simulink model "ASKV3"  (R2024b)
settings: Solver=VariableStepAuto  StartTime=0.0  StopTime=1  RelTol=1e-3
libraries: simulink_extras x3, simulink x3, dspfdesign x1, dspvision x1
settings Model: LastModifiedBy=fredy

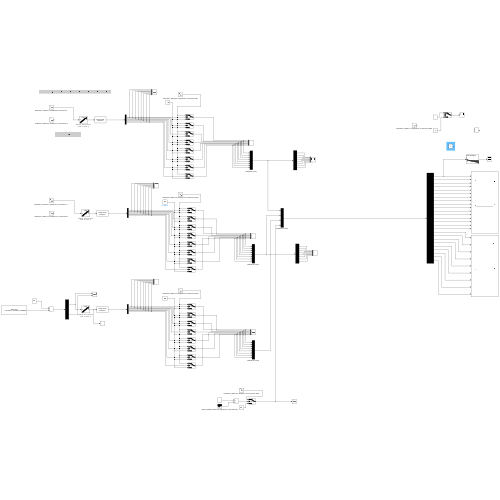
[thumbnail: Simulink's stored preview of the top-level diagram]
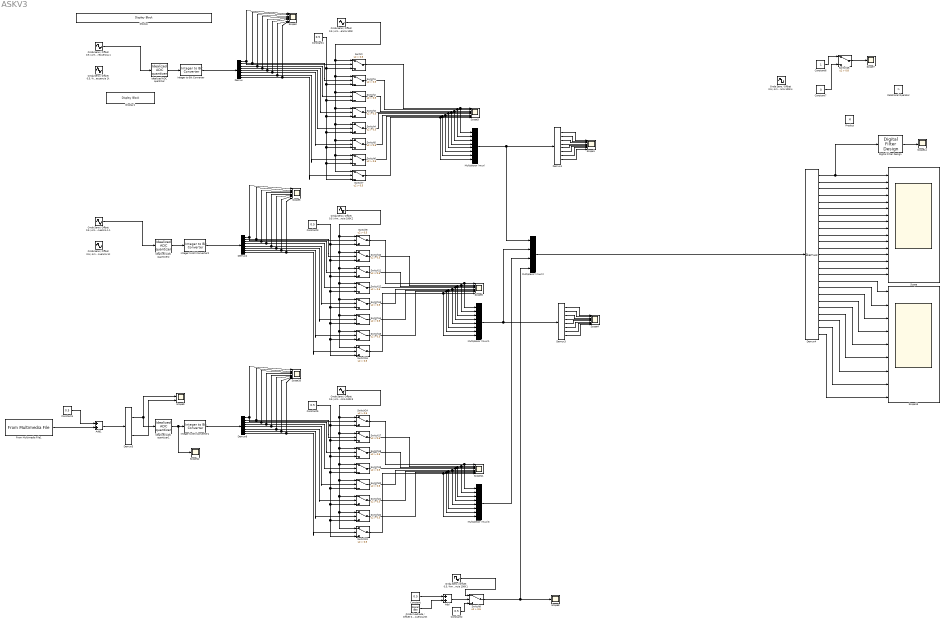
== system ASKV3 ==
  Add : Sum
  Add1 : Sum
  Constant{,1..5} (6 alike) : Constant  Value=0.5
  Constant6 : Constant
  Constant7 : Constant  Value=0
  Demux{,1..3,6} (5 alike) : Demux  Outputs=8
  Demux4 : Demux  Outputs=25
  Demux5 : Demux  Outputs=2
  Digital Filter Design : dspfdesign/Digital Filter Design  mwdsp_browser_bugfix_var=off
  Display : DisplayBlock  LabelPosition=Hide  Transparency=1  Layout=Fill available space
  Display1 : DisplayBlock  LabelPosition=Hide  Transparency=1
  From Multimedia File1 : dspvision/From Multimedia File  inputFilename=D:\Datos Fredy\Programacion\Matlab\Modulacion ASK\audio.mp3  readRange=[1 Inf]  loop=on  numPlays=inf  outputStreams=Audio only  videoDataType=single  audioDataType=single  inheritSampleTime=on  userDefinedSampleTime=1/30  noAudioOutput=off  isIntensityVideo=off  fourcc=RGB  colorVideoFormat=Separate color signals  outputEOF=off  dataOrg=Column-major  audioFrameSize=1  computeAudioFrameSize=off  outSamplingMode=Sample based
      settings: LibrarySourceBlock=audiosources/From Multimedia File
  Idealized ADC quantizer : simulink_extras/Additional Discrete/Idealized ADC quantizer  NumberOfConverterBits=8  Vmin=0  Vmax=1  OutputDataType=double  OutputNegativeValues=off
  Idealized ADC quantizer1 : simulink_extras/Additional Discrete/Idealized ADC quantizer  NumberOfConverterBits=8  Vmin=0  Vmax=1  OutputDataType=double  OutputNegativeValues=off
  Idealized ADC quantizer2 : simulink_extras/Additional Discrete/Idealized ADC quantizer  NumberOfConverterBits=8  Vmin=0  Vmax=1  OutputDataType=double  OutputNegativeValues=off
  Integer to Bit Converter : simulink/Logic and Bit Operations/Integer to Bit Converter  nbits=8  signedInputValues=Unsigned  bitOrder=MSB first  outDtype=Inherit via internal rule
  Integer to Bit Converter1 : simulink/Logic and Bit Operations/Integer to Bit Converter  nbits=8  signedInputValues=Unsigned  bitOrder=MSB first  outDtype=Inherit via internal rule
  Integer to Bit Converter2 : simulink/Logic and Bit Operations/Integer to Bit Converter  nbits=8  signedInputValues=Unsigned  bitOrder=MSB first  outDtype=Inherit via internal rule
  Multiplexor (mux) : Mux  Inputs=8
  Multiplexor (mux)1 : Mux  Inputs=8
  Multiplexor (mux)2 : Mux
  Multiplexor (mux)3 : Mux  Inputs=8
  Onda Cuadrada / Offset 0.5 / Amplitud 0.5 / Frecuencia 5K : SignalGenerator  WaveForm=square  Amplitude=0.5  Frequency=5000
  Onda Seno / Offset 0.5 / Amplitud 0.5 / Frecuencia 1 : Sin  Amplitude=0.5  Bias=0.5  Frequency=6.28321853071  SampleTime=0
  Onda Seno / Offset 0.5 / Amplitud 0.5 / Frecuencia 1.1 : Sin  Amplitude=0.5  Bias=0.5  Frequency=6.28321853071  SampleTime=0
  Onda Seno / Offset 0.5 / Amplitud 0.5 / Frecuencia 100K{,1..4} (5 alike) : Sin  Amplitude=0.5  Bias=0.5  Frequency=628318.5307  SampleTime=0
  Onda Seno / Offset 0.5 / Amplitud 0.5 / Frecuencia 1K : Sin  Amplitude=0.5  Bias=0.5  Frequency=6283.185307  SampleTime=0
  Onda Seno / Offset 0.5 / Amplitud 0.5 / Frecuencia 1k : Sin  Amplitude=0.5  Bias=0.5  Frequency=628321.853071  SampleTime=0
  Product : Product
  Relational Operator : RelationalOperator  Operator=>  OutDataTypeStr=boolean  RndMeth=Simplest  InputSameDT=off
  Scope : Scope  NumInputPorts=16
  Scope{1..6,10..11} (8 alike) : Scope  NumInputPorts=8
  Scope{7..8,12,14} (4 alike) : Scope
  Scope13 : Scope  NumInputPorts=9
  Scope9 : Scope  NumInputPorts=2
  Switch{,1..24} (25 alike) : Switch  Criteria=u2 > Threshold  Threshold=0.5  SaturateOnIntegerOverflow=off  InputSameDT=off
  Switch25 : Switch  Criteria=u2 > Threshold  Threshold=0.8  SaturateOnIntegerOverflow=off  InputSameDT=off
  wires:
  Constant/1 -> Add/1
  Onda Cuadrada / Offset 0.5 / Amplitud 0.5 / Frecuencia 5K/1 -> Add/2
  Add/1 -> Switch8/2
  Idealized ADC quantizer/1 -> Integer to Bit Converter/1
  Onda Seno / Offset 0.5 / Amplitud 0.5 / Frecuencia 100K/1 -> Switch1/1, Switch2/1, Switch7/1, Switch6/1, Switch5/1, Switch4/1, Switch3/1, Switch/1
  Constant1/1 -> Switch/3, Switch1/3, Switch2/3, Switch6/3, Switch7/3, Switch5/3, Switch4/3, Switch3/3
  Idealized ADC quantizer2/1 -> Integer to Bit Converter2/1
  Integer to Bit Converter2/1 -> Demux2/1
  Demux/1 -> Switch/2, Scope2/1
  Integer to Bit Converter/1 -> Demux/1
  Onda Seno / Offset 0.5 / Amplitud 0.5 / Frecuencia 1/1 -> Idealized ADC quantizer/1
  Demux/2 -> Switch1/2, Scope2/2
  Demux/3 -> Switch2/2, Scope2/3
  Demux/5 -> Switch4/2, Scope2/5
  Demux/4 -> Switch3/2, Scope2/4
  Demux/6 -> Switch5/2, Scope2/6
  Demux/7 -> Switch6/2, Scope2/7
  Demux/8 -> Switch7/2, Scope2/8
  Switch1/1 -> Multiplexor (mux)/2, Scope3/2
  Switch2/1 -> Multiplexor (mux)/3, Scope3/3
  Switch3/1 -> Multiplexor (mux)/4, Scope3/4
  Switch4/1 -> Multiplexor (mux)/5, Scope3/5
  Switch5/1 -> Multiplexor (mux)/6, Scope3/6
  Switch6/1 -> Multiplexor (mux)/7, Scope3/7
  Switch7/1 -> Multiplexor (mux)/8, Scope3/8
  Switch/1 -> Multiplexor (mux)/1, Scope3/1
  Multiplexor (mux)/1 -> Multiplexor (mux)2/1, Demux1/1
  Demux1/1 -> Scope1/1
  Demux1/2 -> Scope1/2
  Demux1/3 -> Scope1/3
  Demux1/4 -> Scope1/4
  Demux1/5 -> Scope1/5
  Demux1/6 -> Scope1/6
  Demux1/7 -> Scope1/7
  Demux1/8 -> Scope1/8
  Constant2/1 -> Switch8/3
  Onda Seno / Offset 0.5 / Amplitud 0.5 / Frecuencia 100K1/1 -> Switch8/1
  Switch14/1 -> Multiplexor (mux)1/6, Scope6/6
  Switch15/1 -> Multiplexor (mux)1/7, Scope6/7
  Demux2/7 -> Switch15/2, Scope5/7
  Switch11/1 -> Multiplexor (mux)1/3, Scope6/3
  Demux2/3 -> Switch11/2, Scope5/3
  Demux2/6 -> Switch14/2, Scope5/6
  Demux2/5 -> Switch13/2, Scope5/5
  Demux2/8 -> Switch16/2, Scope5/8
  Onda Seno / Offset 0.5 / Amplitud 0.5 / Frecuencia 100K2/1 -> Switch10/1, Switch11/1, Switch16/1, Switch15/1, Switch14/1, Switch13/1, Switch12/1, Switch9/1
  Demux2/4 -> Switch12/2, Scope5/4
  Demux2/1 -> Switch9/2, Scope5/1
  Switch9/1 -> Multiplexor (mux)1/1, Scope6/1
  Demux3/5 -> Scope4/5
  Constant3/1 -> Switch10/3, Switch11/3, Switch15/3, Switch16/3, Switch14/3, Switch13/3, Switch12/3, Switch9/3
  Demux3/8 -> Scope4/8
  Demux3/1 -> Scope4/1
  Switch10/1 -> Multiplexor (mux)1/2, Scope6/2
  Switch16/1 -> Multiplexor (mux)1/8, Scope6/8
  Switch13/1 -> Multiplexor (mux)1/5, Scope6/5
  Switch12/1 -> Multiplexor (mux)1/4, Scope6/4
  Demux3/6 -> Scope4/6
  Demux3/3 -> Scope4/3
  Demux3/2 -> Scope4/2
  Demux2/2 -> Switch10/2, Scope5/2
  Demux3/4 -> Scope4/4
  Demux3/7 -> Scope4/7
  Multiplexor (mux)2/1 -> Demux4/1
  Demux4/2 -> Scope/2
  Demux4/3 -> Scope/3
  Demux4/4 -> Scope/4
  Demux4/5 -> Scope/5
  Demux4/6 -> Scope/6
  Demux4/7 -> Scope/7
  Demux4/8 -> Scope/8
  Demux4/9 -> Scope/9
  Demux4/10 -> Scope/10
  Demux4/11 -> Scope/11
  Demux4/12 -> Scope/12
  Demux4/13 -> Scope/13
  Demux4/14 -> Scope/14
  Demux4/15 -> Scope/15
  Demux4/16 -> Scope/16
  Onda Seno / Offset 0.5 / Amplitud 0.5 / Frecuencia 1.1/1 -> Idealized ADC quantizer2/1
  Multiplexor (mux)1/1 -> Demux3/1, Multiplexor (mux)2/2
  Switch8/1 -> Multiplexor (mux)2/4, Scope8/1
  Constant4/1 -> Add1/1
  From Multimedia File1/1 -> Add1/2
  Add1/1 -> Demux5/1
  Switch19/1 -> Multiplexor (mux)3/4, Scope11/4
  Switch22/1 -> Multiplexor (mux)3/7, Scope11/7
  Switch20/1 -> Multiplexor (mux)3/5, Scope11/5
  Demux6/6 -> Switch21/2, Scope10/6
  Demux6/1 -> Switch24/2, Scope10/1
  Switch23/1 -> Multiplexor (mux)3/8, Scope11/8
  Demux6/5 -> Switch20/2, Scope10/5
  Onda Seno / Offset 0.5 / Amplitud 0.5 / Frecuencia 100K3/1 -> Switch17/1, Switch18/1, Switch23/1, Switch22/1, Switch21/1, Switch20/1, Switch19/1, Switch24/1
  Demux6/7 -> Switch22/2, Scope10/7
  Demux6/3 -> Switch18/2, Scope10/3
  Demux6/2 -> Switch17/2, Scope10/2
  Switch18/1 -> Multiplexor (mux)3/3, Scope11/3
  Demux6/8 -> Switch23/2, Scope10/8
  Switch17/1 -> Multiplexor (mux)3/2, Scope11/2
  Switch24/1 -> Multiplexor (mux)3/1, Scope11/1
  Constant5/1 -> Switch17/3, Switch18/3, Switch22/3, Switch23/3, Switch21/3, Switch20/3, Switch19/3, Switch24/3
  Idealized ADC quantizer1/1 -> Scope12/1, Integer to Bit Converter1/1
  Demux6/4 -> Switch19/2, Scope10/4
  Integer to Bit Converter1/1 -> Demux6/1
  Switch21/1 -> Multiplexor (mux)3/6, Scope11/6
  Demux5/1 -> Scope9/1, Idealized ADC quantizer1/1
  Demux5/2 -> Scope9/2
  Demux4/17 -> Scope13/1
  Demux4/18 -> Scope13/2
  Demux4/19 -> Scope13/3
  Demux4/20 -> Scope13/4
  Demux4/21 -> Scope13/5
  Demux4/22 -> Scope13/6
  Demux4/23 -> Scope13/7
  Demux4/24 -> Scope13/8
  Demux4/25 -> Scope13/9
  Multiplexor (mux)3/1 -> Multiplexor (mux)2/3
  Constant6/1 -> Switch25/1
  Constant7/1 -> Switch25/3
  Switch25/1 -> Scope7/1
  Demux4/1 -> Digital Filter Design/1, Scope/1
  Digital Filter Design/1 -> Scope14/1
